simulink model "test1"  (R2015a)
settings: Solver=ode45  SolverMode=SingleTasking  StartTime=0.0  StopTime=50  RelTol=1e-3
undefined symbols (not defined in the file): A, B, C, D, G, K1, K2, K_OF, K_SF
settings Model: CovMetricSettings=dwe  CovHtmlReporting=off  covSaveCumulativeToWorkspaceVar=off  CovSaveSingleToWorkspaceVar=off  CovExternalEMLEnable=on  Creator=10911  LastModifiedBy=10911
settings DataIOCC: LimitDataPoints=off  SaveFormat=Dataset  ReturnWorkspaceOutputs=on
settings DebuggingCC: SFUnexpectedBacktrackingDiag=error  SFNoUnconditionalDefaultTransitionDiag=error
settings HardwareCC: ProdBitPerPointer=64  ProdLargestAtomicFloat=Float  ProdIntDivRoundTo=Zero  ProdEndianess=LittleEndian  ProdHWDeviceType=Specified
settings ModelReferenceCC: PropagateSignalLabelsOutOfModel=on
settings SFSimCC: SimUseLocalCustomCode=on
settings RTWCC: RTWUseLocalCustomCode=on
settings GRTTargetCC: TargetLangStandard=C99 (ISO)

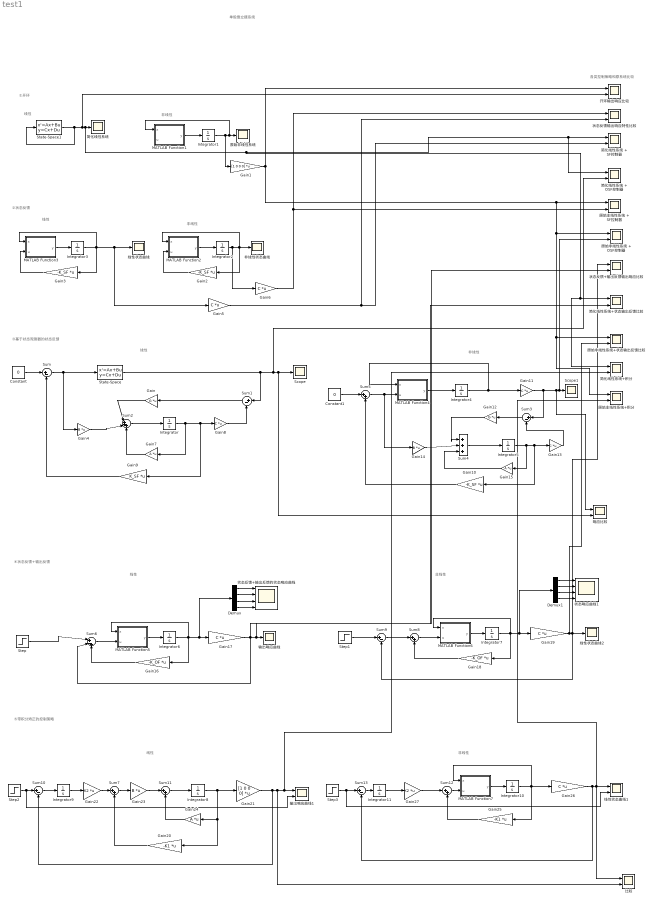
== system test1 ==
  note: 线性
  note: 非线性
  note: ①开环
  note: 非线性
  note: 线性
  note: ②状态反馈
  note: ③基于状态观测器的状态反馈
  note: 非线性
  note: 线性
  note: 非线性
  note: 线性
  note: ④状态反馈+输出反馈
  note: 单级倒立摆系统
  note: ⑤带积分矫正的控制策略
  note: 线性
  note: 非线性
  note: 各类控制策略和原系统比较
  Constant : Constant  Value=0
  Constant1 : Constant  Value=0
  Demux : Demux
  Demux1 : Demux
  Gain : Gain  Gain=G  Multiplication=Matrix(K*u)
  Gain1 : Gain  Gain=[1 0 0 0]  Multiplication=Matrix(K*u)
  Gain10 : Gain  Gain=-K_SF  Multiplication=Matrix(K*u)
  Gain{5..6,8,11,13,17,19,26} (8 alike) : Gain  Gain=C  Multiplication=Matrix(K*u)
  Gain12 : Gain  Gain=G  Multiplication=Matrix(K*u)
  Gain14 : Gain  Gain=B  Multiplication=Matrix(K*u)
  Gain15 : Gain  Gain=A  Multiplication=Matrix(K*u)
  Gain16 : Gain  Gain=-K_OF  Multiplication=Matrix(K*u)
  Gain18 : Gain  Gain=-K_OF  Multiplication=Matrix(K*u)
  Gain2 : Gain  Gain=-K_SF  Multiplication=Matrix(K*u)
  Gain20 : Gain  Gain=-K1  Multiplication=Matrix(K*u)
  Gain21 : Gain  Gain=[1 0 0 0]  Multiplication=Matrix(K*u)
  Gain22 : Gain  Gain=K2  Multiplication=Matrix(K*u)
  Gain23 : Gain  Gain=B  Multiplication=Matrix(K*u)
  Gain24 : Gain  Gain=A  Multiplication=Matrix(K*u)
  Gain25 : Gain  Gain=-K1  Multiplication=Matrix(K*u)
  Gain27 : Gain  Gain=K2  Multiplication=Matrix(K*u)
  Gain3 : Gain  Gain=-K_SF  Multiplication=Matrix(K*u)
  Gain4 : Gain  Gain=B  Multiplication=Matrix(K*u)
  Gain7 : Gain  Gain=A  Multiplication=Matrix(K*u)
  Gain9 : Gain  Gain=K_SF  Multiplication=Matrix(K*u)
  Integrator : Integrator  InitialCondition=[0;0;0.1;0]
  Integrator1 : Integrator  InitialCondition=[1,1,1,1]
  Integrator10 : Integrator  InitialCondition=[0.1 0.1 0.1 0.1]
  Integrator11 : Integrator
  Integrator2 : Integrator  InitialCondition=[0,0,0.3,0]
  Integrator3 : Integrator  InitialCondition=[0;0;0.1;0]
  Integrator4 : Integrator  InitialCondition=[0 0 0.1 0]
  Integrator5 : Integrator  InitialCondition=[0 0 0.1 0]
  Integrator6 : Integrator  InitialCondition=[0.1;0.1;0.1;0.1]
  Integrator7 : Integrator  InitialCondition=[0 0 0.1 0]
  Integrator8 : Integrator
  Integrator9 : Integrator
  MATLAB Function1 : MATLAB Function  TreatAsAtomicUnit=on
      settings: PermitHierarchicalResolution=ParametersOnly
  MATLAB Function2 : MATLAB Function  TreatAsAtomicUnit=on
      settings: PermitHierarchicalResolution=ParametersOnly
  MATLAB Function3 : MATLAB Function  TreatAsAtomicUnit=on
      settings: PermitHierarchicalResolution=ParametersOnly
  MATLAB Function4 : MATLAB Function  TreatAsAtomicUnit=on
      settings: PermitHierarchicalResolution=ParametersOnly
  MATLAB Function5 : MATLAB Function  TreatAsAtomicUnit=on
      settings: PermitHierarchicalResolution=ParametersOnly
  MATLAB Function6 : MATLAB Function  TreatAsAtomicUnit=on
      settings: PermitHierarchicalResolution=ParametersOnly
  MATLAB Function7 : MATLAB Function  TreatAsAtomicUnit=on
      settings: PermitHierarchicalResolution=ParametersOnly
  Scope : Scope
      settings: TimeRange=auto  ShowLegends=on  MaxDataPoints=5000  SaveToWorkspace=off  SaveName=ScopeData4  YMin=-0.06616  YMax=0.59546  SampleTime=-1
  Scope1 : Scope
      settings: TimeRange=auto  ShowLegends=on  MaxDataPoints=5000  SaveToWorkspace=off  SaveName=ScopeData5  YMin=-0.06692  YMax=0.60197  SampleTime=-1
  State-Space : StateSpace  A=A  B=B  C=C  D=D  X0=[0;0;0.1;0]
  State-Space1 : StateSpace  A=[0 1 0 0;0 0 -1 0;0 0 0 1;0 0 22 0]  B=[0;1;0;-2]  C=[1 0 0 0]  D=[0]  X0=1
  Step{,1..3} (4 alike) : Step  SampleTime=0
  Sum{,1,3,9..10,13} (6 alike) : Sum  Inputs=|+-
  Sum{5,7..8,11..12} (5 alike) : Sum  Inputs=|++
  Sum2 : Sum  Inputs=|+++
  Sum4 : Sum  Inputs=|+++
  Sum6 : Sum  Inputs=|+-+
  "原始非线性系统 " : Scope
      settings: TimeRange=auto  MaxDataPoints=5000  SaveToWorkspace=off  SaveName=ScopeData3  YMin=-2.24151  YMax=9.04986  SampleTime=-1
  原始非线性系统 + OSF控制器 : Scope  NumInputPorts=2
      settings: TimeRange=auto  ShowLegends=on  MaxDataPoints=5000  SaveToWorkspace=off  SaveName=ScopeData10  YMin=-5.70884~-0.06691  YMax=61.37957~0.60184  SampleTime=-1
  原始非线性系统 + SF控制器 : Scope  NumInputPorts=2
      settings: TimeRange=auto  ShowLegends=on  MaxDataPoints=5000  SaveToWorkspace=off  SaveName=ScopeData9  YMin=-5.70884~-0.22645  YMax=61.37957~1.83173  SampleTime=-1
  原始非线性系统+状态输出反馈比较 : Scope  NumInputPorts=2
      settings: TimeRange=auto  ShowLegends=on  MaxDataPoints=5000  SaveToWorkspace=off  SaveName=ScopeData17  YMin=-5.70884~-0.2719  YMax=61.37957~0.2083  SampleTime=-1
  原始非线性系统+积分 : Scope  NumInputPorts=2
      settings: TimeRange=auto  ShowLegends=on  MaxDataPoints=5000  SaveName=ScopeData22  YMin=-5.81748~-0.3525  YMax=62.35734~1.21224  SampleTime=-1
  响应比较 : Scope  NumInputPorts=2
      settings: TimeRange=auto  ShowLegends=on  MaxDataPoints=5000  SaveToWorkspace=off  SaveName=ScopeData6  YMin=-0.06691~-0.06612  YMax=0.60184~0.59505  SampleTime=-1
  开环输出响应比较 : Scope  NumInputPorts=2
      settings: TimeRange=auto  ShowLegends=on  MaxDataPoints=5000  SaveName=ScopeData4  YMin=-5.70884~-34377419029095608970641659881482028377840226357392472077060944427337011146029719643187965309510221824.00000  YMax=61.37957~3819713225455066638107157978807660167821796549519740613958717658852698355546752598154734509418872832.00000  SampleTime=-1
  比较 : Scope  NumInputPorts=2
      settings: TimeRange=auto  ShowLegends=on  MaxDataPoints=5000  SaveName=ScopeData20  YMin=-0.44699~-0.44699  YMax=1.38767~1.38767  SampleTime=-1
  状态反馈+输出反馈的状态响应曲线 : Scope  NumInputPorts=4
      settings: TimeRange=auto  ShowLegends=on  MaxDataPoints=5000  SaveName=ScopeData13  YMin=-0.30317~-0.55497~-0.11586~-0.63266  YMax=0.40493~0.6926~0.12444~0.25546  SampleTime=-1
  状态反馈+输出反馈输出响应比较 : Scope  NumInputPorts=2
      settings: TimeRange=auto  ShowLegends=on  MaxDataPoints=5000  SaveToWorkspace=off  SaveName=ScopeData15  YMin=-0.2719~-0.30317  YMax=0.2083~0.40493  SampleTime=-1
  状态反馈输出响应特性比较 : Scope  NumInputPorts=2
      settings: TimeRange=auto  ShowLegends=on  MaxDataPoints=5000  YMin=-0.22648~-0.06616  YMax=1.83214~0.5954  SampleTime=-1
  状态响应曲线1 : Scope  NumInputPorts=4
      settings: TimeRange=auto  ShowLegends=on  MaxDataPoints=5000  SaveName=ScopeData14  YMin=-0.27136~-0.39416~-0.06684~-0.45067  YMax=0.20836~0.43292~0.11854~0.15007  SampleTime=-1
  简化线性系统 : Scope
      settings: TimeRange=auto  ShowLegends=on  MaxDataPoints=5000  SaveToWorkspace=off  SaveName=ScopeData2  YMin=-34384161405055965491691081453823166918554485539591660952149503870416325472888531861639677464440471552.00000  YMax=3820462378339550642038513369464201369027216824666347526679478734413191023758498129679805715377553408.00000  SampleTime=-1
  简化线性系统 + OSF控制器 : Scope  NumInputPorts=2
      settings: TimeRange=auto  ShowLegends=on  MaxDataPoints=5000  SaveToWorkspace=off  SaveName=ScopeData8  YMin=-34377419029095608970641659881482028377840226357392472077060944427337011146029719643187965309510221824.00000~-0.06612  YMax=3819713225455066638107157978807660167821796549519740613958717658852698355546752598154734509418872832.00000~0.59505  SampleTime=-1
  简化线性系统 + SF控制器 : Scope  NumInputPorts=2
      settings: TimeRange=auto  ShowLegends=on  MaxDataPoints=5000  SaveToWorkspace=off  SaveName=ScopeData7  YMin=-34377419029095608970641659881482028377840226357392472077060944427337011146029719643187965309510221824.00000~-0.06612  YMax=3819713225455066638107157978807660167821796549519740613958717658852698355546752598154734509418872832.00000~0.59505  SampleTime=-1
  简化线性系统+状态输出反馈比较 : Scope  NumInputPorts=2
      settings: TimeRange=auto  ShowLegends=on  MaxDataPoints=5000  SaveToWorkspace=off  SaveName=ScopeData16  YMin=-34377419029095608970641659881482028377840226357392472077060944427337011146029719643187965309510221824.00000~-0.30317  YMax=3819713225455066638107157978807660167821796549519740613958717658852698355546752598154734509418872832.00000~0.40493  SampleTime=-1
  简化线性系统+积分 : Scope  NumInputPorts=2
      settings: TimeRange=auto  ShowLegends=on  MaxDataPoints=5000  SaveName=ScopeData21  YMin=-34384161405055965491691081453823166918554485539591660952149503870416325472888531861639677464440471552.00000~-0.18895  YMax=3820462378339550642038513369464201369027216824666347526679478734413191023758498129679805715377553408.00000~1.18353  SampleTime=-1
  线性状态曲线 : Scope
      settings: TimeRange=auto  MaxDataPoints=5000  SaveName=ScopeData3  YMin=-0.3363  YMax=0.62507  SampleTime=-1
  线性状态曲线1 : Scope  NumInputPorts=2
      settings: TimeRange=auto  MaxDataPoints=5000  SaveName=ScopeData18  YMin=-0.44699~-5  YMax=1.38767~5  SampleTime=-1
  线性状态曲线2 : Scope
      settings: TimeRange=auto  MaxDataPoints=5000  SaveName=ScopeData12  YMin=-6169.89092  YMax=3862.2887  SampleTime=-1
  输出响应曲线 : Scope
      settings: TimeRange=auto  MaxDataPoints=5000  SaveName=ScopeData11  YMin=-0.30281  YMax=0.40555  SampleTime=-1
  输出响应曲线1 : Scope  NumInputPorts=2
      settings: TimeRange=auto  MaxDataPoints=5000  SaveName=ScopeData19  YMin=-0.20186~-5  YMax=1.31723~5  SampleTime=-1
  非线性状态曲线 : Scope
      settings: TimeRange=auto  MaxDataPoints=5000  SaveName=ScopeData2  YMin=-0.96496  YMax=1.90088  SampleTime=-1
  wires:
  Integrator1/1 -> Gain1/1, MATLAB Function1/1(x), "原始非线性系统 "/1
  Gain1/1 -> 原始非线性系统 + OSF控制器/1, 原始非线性系统+积分/1, 原始非线性系统+状态输出反馈比较/1, 原始非线性系统 + SF控制器/1, 开环输出响应比较/1
  MATLAB Function1/1(y) -> Integrator1/1
  State-Space1/1 -> 开环输出响应比较/2, 简化线性系统+积分/1, 简化线性系统+状态输出反馈比较/1, 简化线性系统 + OSF控制器/1, 简化线性系统 + SF控制器/1, 简化线性系统/1, State-Space1/1
  Gain6/1 -> 原始非线性系统 + SF控制器/2, 状态反馈输出响应特性比较/1
  MATLAB Function3/1(y) -> Integrator3/1
  Integrator3/1 -> Gain3/1, MATLAB Function3/1(x), Gain5/1, 线性状态曲线/1
  Gain2/1 -> MATLAB Function2/2(u)
  Integrator2/1 -> Gain6/1, Gain2/1, MATLAB Function2/1(x), 非线性状态曲线/1
  MATLAB Function2/1(y) -> Integrator2/1
  Gain3/1 -> MATLAB Function3/2(u)
  Gain5/1 -> 简化线性系统 + SF控制器/2, 状态反馈输出响应特性比较/2
  MATLAB Function4/1(y) -> Integrator4/1
  Integrator5/1 -> Gain10/1, Gain13/1, Gain15/1
  Gain14/1 -> Sum4/2
  Sum3/1 -> Gain12/1
  Gain15/1 -> Sum4/3
  Gain13/1 -> Sum3/2
  Integrator4/1 -> MATLAB Function4/1(x), Gain11/1
  Gain12/1 -> Sum4/1
  Sum4/1 -> Integrator5/1
  Constant/1 -> Sum/1
  Gain11/1 -> Sum3/1, 响应比较/1, 原始非线性系统 + OSF控制器/2, Scope1/1
  Gain10/1 -> Sum5/2
  State-Space/1 -> Sum1/1, 简化线性系统 + OSF控制器/2, 响应比较/2, Scope/1
  Integrator/1 -> Gain9/1, Gain8/1, Gain7/1
  Gain/1 -> Sum2/1
  Gain8/1 -> Sum1/2
  Sum2/1 -> Integrator/1
  Gain7/1 -> Sum2/3
  Gain4/1 -> Sum2/2
  Sum1/1 -> Gain/1
  Constant1/1 -> Sum5/1
  Gain9/1 -> Sum/2
  Sum5/1 -> Gain14/1, MATLAB Function4/2(u)
  Sum/1 -> Gain4/1, State-Space/1
  MATLAB Function5/1(y) -> Integrator6/1
  Sum6/1 -> MATLAB Function5/2(u)
  Integrator6/1 -> MATLAB Function5/1(x), Demux/1, Gain17/1, Gain16/1
  Gain17/1 -> Sum6/2, 简化线性系统+状态输出反馈比较/2, 输出响应曲线/1, 状态反馈+输出反馈输出响应比较/2
  Step/1 -> Sum6/1
  Gain19/1 -> 原始非线性系统+状态输出反馈比较/2, Sum9/2, 状态反馈+输出反馈输出响应比较/1, 线性状态曲线2/1
  MATLAB Function6/1(y) -> Integrator7/1
  Step1/1 -> Sum9/1
  Sum9/1 -> Sum8/1
  Gain18/1 -> Sum8/2
  Sum8/1 -> MATLAB Function6/2(u)
  Gain16/1 -> Sum6/3
  Demux/1 -> 状态反馈+输出反馈的状态响应曲线/1
  Demux/2 -> 状态反馈+输出反馈的状态响应曲线/2
  Demux/3 -> 状态反馈+输出反馈的状态响应曲线/3
  Demux/4 -> 状态反馈+输出反馈的状态响应曲线/4
  Integrator7/1 -> MATLAB Function6/1(x), Demux1/1, Gain19/1, Gain18/1
  Demux1/2 -> 状态响应曲线1/2
  Demux1/4 -> 状态响应曲线1/4
  Demux1/3 -> 状态响应曲线1/3
  Demux1/1 -> 状态响应曲线1/1
  Gain21/1 -> Sum10/2, 比较/2, 简化线性系统+积分/2, 输出响应曲线1/1
  Integrator8/1 -> Gain24/1, Gain20/1, Gain21/1
  Sum11/1 -> Integrator8/1
  Sum7/1 -> Gain23/1
  Gain20/1 -> Sum7/2
  Step2/1 -> 输出响应曲线1/2, Sum10/1
  Sum10/1 -> Integrator9/1
  Integrator9/1 -> Gain22/1
  Gain22/1 -> Sum7/1
  Gain24/1 -> Sum11/2
  Gain23/1 -> Sum11/1
  Sum12/1 -> MATLAB Function7/2(u)
  MATLAB Function7/1(y) -> Integrator10/1
  Step3/1 -> 线性状态曲线1/2, Sum13/1
  Gain26/1 -> Sum13/2, 原始非线性系统+积分/2, 线性状态曲线1/1, 比较/1
  Integrator10/1 -> MATLAB Function7/1(x), Gain26/1, Gain25/1
  Gain25/1 -> Sum12/2
  Sum13/1 -> Integrator11/1
  Integrator11/1 -> Gain27/1
  Gain27/1 -> Sum12/1

== matlab function test1/MATLAB Function1 ==
  data: x input; y output; u input
function y = fcn(x,u)

M = 1;
m = 0.1;
l = 0.5;
g = 9.8;

dx1 = x(2);
dx2 = (u+m*l*sin(x(3)*x(4)*x(4))-m*g*cos(x(3))*sin(x(3)))/(M + m - m*cos(x(3))*cos(x(3)));
dx3 = x(4);
dx4 = (u*cos(x(3))-(M+m)*g*sin(x(3))+m*l*sin(x(3))*cos(x(3)*x(4)*x(4)))/(m*l*cos(x(3))*cos(x(3))-(M+m)*l);
y = [dx1;dx2;dx3;dx4];

== matlab function test1/MATLAB Function2 ==
  data: x input; y output; u input
function y = fcn(x,u)
M = 1;
m = 0.1;
l = 0.5;
g = 9.8;
x1=x(1);
x2=x(2);
x3=x(3);
x4=x(4);

dx1 = x2;
dx2 =(u + m*l*x4*x4*sin(x3) - m*g*sin(x3)*cos(x3))/(M + m - m*cos(x3)*cos(x3));
dx3 = x4;
dx4 =(-u*cos(x3) + (M+m)*g*sin(x3) - m*l*x4*x4*sin(x3)*cos(x3))/((M+m)*l - m*l*cos(x3)*cos(x3));
y = [dx1;dx2;dx3;dx4];

== matlab function test1/MATLAB Function3 ==
  data: x input; y output; u input
function y = fcn(x,u)

dx1 = x(2);
dx2 = -x(3)+u;
dx3 = x(4);
dx4 = 22*x(3)-2*u;

y = [dx1;dx2;dx3;dx4];

== matlab function test1/MATLAB Function4 ==
  data: x input; y output; u input
function y = fcn(x,u)
M = 1;
m = 0.1;
l = 0.5;
g = 9.8;
x1=x(1);
x2=x(2);
x3=x(3);
x4=x(4);

dx1 = x2;
dx2 =(u + m*l*x4*x4*sin(x3) - m*g*sin(x3)*cos(x3))/(M + m - m*cos(x3)*cos(x3));
dx3 = x4;
dx4 =(-u*cos(x3) + (M+m)*g*sin(x3) - m*l*x4*x4*sin(x3)*cos(x3))/((M+m)*l - m*l*cos(x3)*cos(x3));
y = [dx1;dx2;dx3;dx4];

== matlab function test1/MATLAB Function5 ==
  data: x input; y output; u input
function y = fcn(x,u)

dx1 = x(2);
dx2 = -x(3)+u;
dx3 = x(4);
dx4 = 22*x(3)-2*u;

y = [dx1;dx2;dx3;dx4];

== matlab function test1/MATLAB Function6 ==
  data: x input; y output; u input
function y = fcn(x,u)
M = 1;
m = 0.1;
l = 0.5;
g = 9.8;
x1=x(1);
x2=x(2);
x3=x(3);
x4=x(4);

dx1 = x2;
dx2 =(u + m*l*x4*x4*sin(x3) - m*g*sin(x3)*cos(x3))/(M + m - m*cos(x3)*cos(x3));
dx3 = x4;
dx4 =(-u*cos(x3) + (M+m)*g*sin(x3) - m*l*x4*x4*sin(x3)*cos(x3))/((M+m)*l - m*l*cos(x3)*cos(x3));
y = [dx1;dx2;dx3;dx4];

== matlab function test1/MATLAB Function7 ==
  data: x input; y output; u input
function y = fcn(x,u)
M = 1;
m = 0.1;
l = 0.5;
g = 9.8;
x1=x(1);
x2=x(2);
x3=x(3);
x4=x(4);

dx1 = x2;
dx2 =(u + m*l*x4*x4*sin(x3) - m*g*sin(x3)*cos(x3))/(M + m - m*cos(x3)*cos(x3));
dx3 = x4;
dx4 =(-u*cos(x3) + (M+m)*g*sin(x3) - m*l*x4*x4*sin(x3)*cos(x3))/((M+m)*l - m*l*cos(x3)*cos(x3));
y = [dx1;dx2;dx3;dx4];
